simulink model "SimulinkLineTracking_without_PID"  (R2019b)
settings: Solver=FixedStepAuto  StartTime=0.0  StopTime=inf  RelTol=1e-3  EnableMultiTasking=on
libraries: legoev3lib x6
settings Model: ExtModeTrigDuration=2  Creator=nikit  LastModifiedBy=nikit
settings SolverCC: PositivePriorityOrder=on
settings OptimizationCC: EnhancedBackFolding=on  PassReuseOutputArgsAs=Individual arguments  ZeroExternalMemoryAtStartup=off  ZeroInternalMemoryAtStartup=off  MaxStackSize=64  OptimizeBlockOrder=speed  DifferentSizesBufferReuse=on  OptimizationCustomize=off  EfficientTunableParamExpr=on
settings DebuggingCC: ParameterTunabilityLossMsg=error
settings HardwareCC: ProdBitPerPointer=32  ProdBitPerSizeT=32  ProdBitPerPtrDiffT=32  ProdLargestAtomicInteger=Long  ProdWordSize=32  ProdHWDeviceType=ARM Compatible->ARM 9
settings SFSimCC: MATLABDynamicMemAlloc=off
settings RTWCC: SystemTargetFile=ert.tlc  HardwareBoard=LEGO MINDSTORMS EV3  TLCOptions="-aInlineSetEventsForThisBaseRateFcn=TLC_FALSE -aSuppressMultiTaskScheduler=TLC_FALSE  -aRateBasedStepFcn=0"  TemplateMakefile=ert_default_tmf  GenerateReport=on  Toolchain=Sourcery G++ Lite v2009q3  IncludeHyperlinkInReport=on  LaunchReport=on  GenerateTraceInfo=on  GenerateTraceReport=on  GenerateTraceReportSl=on  GenerateTraceReportSf=on  GenerateTraceReportEml=on
settings CodeAppCC: ForceParamTrailComments=on  IgnoreCustomStorageClasses=off  OperatorAnnotations=on  SimulinkDataObjDesc=on  SFDataObjDesc=on  InsertBlockDesc=on
settings ERTTargetCC: SupportContinuousTime=on  SupportVariableSizeSignals=on

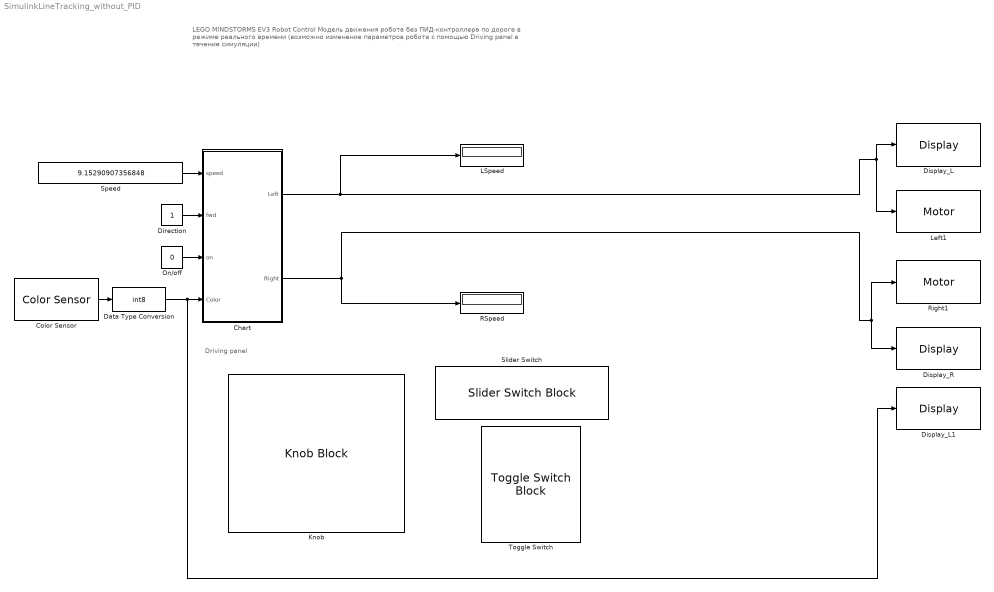
== system SimulinkLineTracking_without_PID ==
  note: Driving panel
  note: LEGO MINDSTORMS EV3 Robot Control
      | Модель движения робота без ПИД-контроллера по дороге в режиме реального времени
      | (возможно изменение параметров робота с помощью Driving panel в течение симуляции)
  Chart : Stateflow chart  TreatAsAtomicUnit=on
  Color Sensor : legoev3lib/Color Sensor  portNumber=2  mode=Color  sampleTime=0.1
      settings: SourceProductName=Simulink Support Package for LEGO MINDSTORMS EV3 Hardware  SourceProductBaseCode=LEGOEV3
  Data Type Conversion : DataTypeConversion  OutDataTypeStr=int8
  Direction : Constant  OutDataTypeStr=int8
  Display_L : legoev3lib/Display  slcdStr=Left  slcdLine=1  slcdFormat=Decimal
      settings: SourceProductName=Simulink Support Package for LEGO MINDSTORMS EV3 Hardware  SourceProductBaseCode=LEGOEV3
  Display_L1 : legoev3lib/Display  slcdStr=Color  slcdLine=3  slcdFormat=Decimal
      settings: SourceProductName=Simulink Support Package for LEGO MINDSTORMS EV3 Hardware  SourceProductBaseCode=LEGOEV3
  Display_R : legoev3lib/Display  slcdStr=Right  slcdLine=2  slcdFormat=Decimal
      settings: SourceProductName=Simulink Support Package for LEGO MINDSTORMS EV3 Hardware  SourceProductBaseCode=LEGOEV3
  Knob : KnobBlock
  LSpeed : Display
  Left1 : legoev3lib/Motor  sportNumber=A  sstopAction=Brake
  On/off : Constant  Value=0  OutDataTypeStr=int8
  RSpeed : Display
  Right1 : legoev3lib/Motor  sportNumber=D  sstopAction=Brake
  Slider Switch : SliderSwitchBlock
      settings: Values={{'Off', 'On'}, [0 1]}
  Speed : Constant  Value=9.15290907356848  OutDataTypeStr=int8
  Toggle Switch : ToggleSwitchBlock
      settings: Values={{'Back', 'Forward'}, [-1 1]}
  wires:
  Chart/1(Left) -> Left1/1, Display_L/1, LSpeed/1
  Chart/2(Right) -> Display_R/1, Right1/1, RSpeed/1
  Direction/1 -> Chart/2(fwd)
  Speed/1 -> Chart/1(speed)
  On/off/1 -> Chart/3(on)
  Color Sensor/1 -> Data Type Conversion/1
  Data Type Conversion/1 -> Display_L1/1, Chart/4(Color)

== stateflow chart SimulinkLineTracking_without_PID/Chart ==
  state Straight
    during:
    Left = speed*fwd*on;
    Right = Left;
  state Left_Diagonal
    during:
    Right = speed*fwd*on;
    Left = 0.6*Right;
  state Right_Diagonal
    during:
    Left = speed*fwd*on;
    Right = 0.6*Left;
  (default) -> Straight
  Straight -> Left_Diagonal [order 1] : [Color<10]
  Straight -> Right_Diagonal [order 2] : [Color>15]
  Left_Diagonal -> Right_Diagonal : [Color>15]
  Right_Diagonal -> Left_Diagonal : [Color<10]
  data: Left output int8 size=1; speed input int8; fwd input int8; on input int8; Color input int8; Right output int8
